simulink model "lab6c_practice"  (R2016b)
settings: Solver=FixedStepAuto  StartTime=0.0  StopTime=inf  FixedStep=0.005  RelTol=1e-3  EnableMultiTasking=on
values from neighbouring files (symbols this model uses):
  A = [0 a12   0   0 ... (first row only)    [Lab6c.m]    (also in Prelab6c.m)
  Bk = B*K    [Lab6c.m]    (also in Prelab6c.m)
  C = [1 0 0 0 ... (first row only)    [Lab6c.m]    (also in Prelab6c.m)
  Cl = L*C    [Lab6c.m]    (also in Prelab6c.m)
  ref = [0.3 0 0 0]    [Lab6c.m]    (also in Prelab6c.m = [0 0 0 0])
  res_a = -1/651.9    (= -0.00153397760393)    [Lab6c.m]
  res_p = 1/43960    (= 2.27479526843e-05)    [Lab6c.m]
undefined symbols (not defined in the file or in its folder): HIL, K
libraries: quarc_library x3
settings Model: SimulationMode=external  Creator=ee105-abq  LastModifiedBy=ee105-abq
settings SolverCC: PositivePriorityOrder=on
settings DataIOCC: SaveFormat=Array
settings RTWCC: SystemTargetFile=quarc_win64.tlc  TemplateMakefile=quarc_default_tmf  Description=QUARC Win64 Target
settings STFCustomTargetCC: TargetPreCompLibLocation=C:\PROGRA~3\QUARC\lib\2016b\win64\release  TargetLangStandard=C99 (ISO)  ConcurrentExecutionCompliant=on  SystemTargetFile=quarc_win64.tlc
settings GRTTargetCC: TargetPreCompLibLocation=C:\PROGRA~3\QUARC\lib\2016b\win64\release  ParMdlRefBuildCompliant=off  CompOptLevelCompliant=off  CombineOutputUpdateFcns=off  MatFileLogging=off  CPPClassGenCompliant=off  GRTInterface=on  UseToolchainInfoCompliant=off  ExtMode=on  ExtModeMexFile=quarc_comm

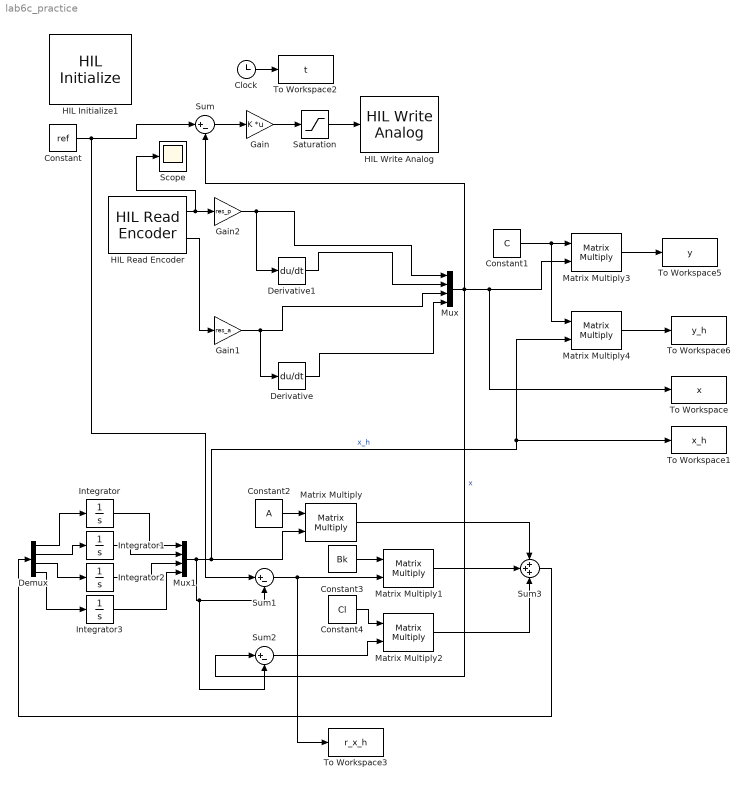
== system lab6c_practice ==
  Clock : Clock
  Constant : Constant  Value=ref
  Constant1 : Constant  Value=C
  Constant2 : Constant  Value=A
  Constant3 : Constant  Value=Bk
  Constant4 : Constant  Value=Cl
  Demux : Demux
  Derivative : Derivative
  Derivative1 : Derivative
  Gain : Gain  Gain=K  Multiplication=Matrix(K*u)
  Gain1 : Gain  Gain=res_a
  Gain2 : Gain  Gain=res_p
  HIL Initialize1 : quarc_library/Data Acquisition/Generic/Configuration/HIL Initialize  object_name=HIL-2  board_type=q4  board_number=0  board_options=""  exclusive=off  active=on  hardware_clocks=[0:1]  clock_modes=[0 0]  initial_clock_frequencies=[]  set_clock_params_at_start=on  set_clock_params_at_switch_in=off  set_clock_frequencies_at_start=off  set_clock_frequencies_at_switch_in=off  analog_input_channels=[0:3]  analog_input_configurations=[]  analog_input_maximums=10  analog_input_minimums=-10  set_analog_input_params_at_start=off  set_analog_input_params_at_switch_in=off  analog_output_channels=[0:3]  analog_output_maximums=[10]  analog_output_minimums=[-10]  initial_analog_outputs=[0]  final_analog_outputs=[0]  watchdog_analog_outputs=0  set_analog_output_params_at_start=on  set_analog_output_params_at_switch_in=off  set_analog_outputs_at_start=on  set_analog_outputs_at_switch_in=off  set_analog_outputs_at_terminate=on  set_analog_outputs_at_switch_out=off  set_analog_outputs_on_watchdog=off  digital_input_channels=[]  digital_output_channels=[]  digital_output_configuration=[]  initial_digital_outputs=[1]  final_digital_outputs=[1]  watchdog_digital_outputs=[2]  set_digital_output_params_at_start=off  set_digital_output_params_at_switch_in=off  set_digital_outputs_at_start=on  set_digital_outputs_at_switch_in=off  set_digital_outputs_at_terminate=on  set_digital_outputs_at_switch_out=off  set_digital_outputs_on_watchdog=off  encoder_channels=[0:3]  quadrature=[4]  encoder_filter_frequency=(1/60e-9)/1  initial_encoder_counts=[0]  set_encoder_params_at_start=on  set_encoder_params_at_switch_in=off  set_encoder_counts_at_start=on  set_encoder_counts_at_switch_in=off  pwm_channels=[]  pwm_modes=[0]  pwm_frequency=(1/60e-9)/1024  pwm_configuration=[]  pwm_alignment=[]  pwm_polarity=[]  pwm_leading_deadband=[]  pwm_trailing_deadband=[]  initial_pwm_outputs=[0]  final_pwm_outputs=[0]  watchdog_pwm_outputs=[]  set_pwm_params_at_start=on  set_pwm_params_at_switch_in=off  set_pwm_outputs_at_start=on  set_pwm_outputs_at_switch_in=off  set_pwm_outputs_at_terminate=on  set_pwm_outputs_at_switch_out=off  set_pwm_outputs_on_watchdog=off  other_output_channels=[]  initial_other_outputs=[]  final_other_outputs=[]  watchdog_other_outputs=[]  set_other_outputs_at_start=off  set_other_outputs_at_switch_in=off  set_other_outputs_at_terminate=off  set_other_outputs_at_switch_out=off  set_other_outputs_on_watchdog=off
  HIL Read Encoder : quarc_library/Data Acquisition/Generic/Immediate I//O/HIL Read Encoder  object_name=HIL-2  channels=[0:1]  sample_time=qc_get_step_size  active=on  vector_output=off  data_type_mode=Inherit via back propagation  data_type=double
  HIL Write Analog : quarc_library/Data Acquisition/Generic/Immediate I//O/HIL Write Analog  object_name=HIL-2  channels=0  sample_time=-1  active=off  vector_input=off
  Integrator{,1..3} (4 alike) : Integrator
  Matrix Multiply{,1..4} (5 alike) : Product  Multiplication=Matrix(*)
  Mux : Mux
  Mux1 : Mux
  Saturation : Saturate  UpperLimit=6  LowerLimit=-6
      settings: LockScale=on
  Scope : Scope
  Sum : Sum  Inputs=|+-
  Sum1 : Sum  Inputs=|+-
  Sum2 : Sum  Inputs=|+-
  Sum3 : Sum  Inputs=+++
  To Workspace : ToWorkspace  VariableName=x  SampleTime=-1
  To Workspace1 : ToWorkspace  VariableName=x_h  SampleTime=-1
  To Workspace2 : ToWorkspace  VariableName=t  SampleTime=-1
  To Workspace3 : ToWorkspace  VariableName=r_x_h  SampleTime=-1
  To Workspace5 : ToWorkspace  VariableName=y  SampleTime=-1
  To Workspace6 : ToWorkspace  VariableName=y_h  SampleTime=-1
  wires:
  Saturation/1 -> HIL Write Analog/1
  Clock/1 -> To Workspace2/1
  Derivative1/1 -> Mux/2
  Derivative/1 -> Mux/4
  HIL Read Encoder/1 -> Scope/1, Gain2/1
  Gain2/1 -> Derivative1/1, Mux/1
  HIL Read Encoder/2 -> Gain1/1
  Gain1/1 -> Derivative/1, Mux/3
  Mux/1 -> To Workspace/1, Matrix Multiply3/2, Sum2/1, Sum/2  "x"
  Gain/1 -> Saturation/1
  Sum/1 -> Gain/1
  Constant/1 -> Sum/1, Sum1/1
  Integrator/1 -> Mux1/1
  Integrator1/1 -> Mux1/2
  Integrator2/1 -> Mux1/3
  Integrator3/1 -> Mux1/4
  Demux/1 -> Integrator/1
  Demux/2 -> Integrator1/1
  Demux/3 -> Integrator2/1
  Demux/4 -> Integrator3/1
  Constant2/1 -> Matrix Multiply/1
  Mux1/1 -> Sum2/2, Sum1/2, Matrix Multiply/2, Matrix Multiply4/2, To Workspace1/1  "x_h"
  Constant3/1 -> Matrix Multiply1/1
  Sum1/1 -> To Workspace3/1, Matrix Multiply1/2
  Constant4/1 -> Matrix Multiply2/1
  Sum2/1 -> Matrix Multiply2/2
  Matrix Multiply1/1 -> Sum3/2
  Matrix Multiply/1 -> Sum3/1
  Matrix Multiply2/1 -> Sum3/3
  Sum3/1 -> Demux/1
  Constant1/1 -> Matrix Multiply4/1, Matrix Multiply3/1
  Matrix Multiply3/1 -> To Workspace5/1
  Matrix Multiply4/1 -> To Workspace6/1
